simulink model "vector2"  (R2020a)
settings: Solver=FixedStepDiscrete  StartTime=0.0  StopTime=10.0  FixedStep=1  RelTol=1e-3
libraries: simulink x5, hdlsllib x3
settings Model: Creator=cyarp  LastModifiedBy=cyarp

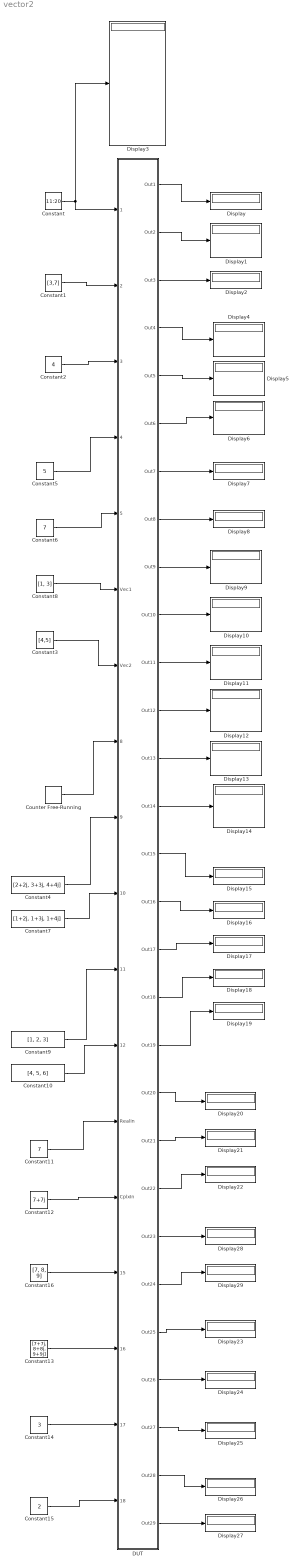
== system vector2 ==
  Constant : Constant  Value=11:20
  Constant1 : Constant  Value=[3,7]  OutDataTypeStr=int8
  Constant10 : Constant  Value=[4, 5, 6]
  Constant11 : Constant  Value=7
  Constant12 : Constant  Value=7+7j
  Constant13 : Constant  Value=[7+7j, 8+8j, 9+9j]
  Constant14 : Constant  Value=3  OutDataTypeStr=int8
  Constant15 : Constant  Value=2  OutDataTypeStr=int8
  Constant16 : Constant  Value=[7, 8, 9]
  Constant2 : Constant  Value=4  OutDataTypeStr=int8
  Constant3 : Constant  Value=[4,5]
  Constant4 : Constant  Value=[2+2j, 3+3j, 4+4j]
  Constant5 : Constant  Value=5
  Constant6 : Constant  Value=7
  Constant7 : Constant  Value=[1+2j, 1+3j, 1+4j]
  Constant8 : Constant  Value=[1, 3]
  Constant9 : Constant  Value=[1, 2, 3]
  Counter Free-Running : simulink/Sources/Counter Free-Running  NumBits=16  tsamp=-1
  DUT : Subsystem
  Display{,1..29} (30 alike) : Display
  wires:
  Constant/1 -> DUT/1(InVector), Display3/1
  Constant1/1 -> DUT/2(VecSelect)
  Constant2/1 -> DUT/3(ScalarSelect)
  Constant5/1 -> DUT/4(Scalar1)
  Constant6/1 -> DUT/5(Scalar2)
  Constant8/1 -> DUT/6(Vec1)
  Constant3/1 -> DUT/7(Vec2)
  Counter Free-Running/1 -> DUT/8(counter)
  Constant4/1 -> DUT/9(ComplVec1)
  Constant7/1 -> DUT/10(ComplVec2)
  Constant9/1 -> DUT/11(RealVec1)
  Constant10/1 -> DUT/12(RealVec2)
  Constant11/1 -> DUT/13(RealIn)
  Constant12/1 -> DUT/14(CplxIn)
  Constant13/1 -> DUT/16(ComplexCoef)
  Constant14/1 -> DUT/17(signed1)
  Constant15/1 -> DUT/18(signed2)
  DUT/1(Out1) -> Display/1
  DUT/2(Out2) -> Display1/1
  DUT/3(Out3) -> Display2/1
  DUT/4(Out4) -> Display4/1
  DUT/5(Out5) -> Display5/1
  DUT/6(Out6) -> Display6/1
  DUT/7(Out7) -> Display7/1
  DUT/8(Out8) -> Display8/1
  DUT/9(Out9) -> Display9/1
  DUT/10(Out10) -> Display10/1
  DUT/11(Out11) -> Display11/1
  DUT/12(Out12) -> Display12/1
  DUT/13(Out13) -> Display13/1
  DUT/14(Out14) -> Display14/1
  DUT/15(Out15) -> Display15/1
  DUT/16(Out16) -> Display16/1
  DUT/17(Out17) -> Display17/1
  DUT/18(Out18) -> Display18/1
  DUT/19(Out19) -> Display19/1
  DUT/20(Out20) -> Display20/1
  DUT/21(Out21) -> Display21/1
  DUT/22(Out22) -> Display22/1
  DUT/25(Out25) -> Display23/1
  DUT/26(Out26) -> Display24/1
  DUT/27(Out27) -> Display25/1
  DUT/28(Out28) -> Display26/1
  DUT/29(Out29) -> Display27/1
  DUT/23(Out23) -> Display28/1
  DUT/24(Out24) -> Display29/1
  Constant16/1 -> DUT/15(RealCoef)

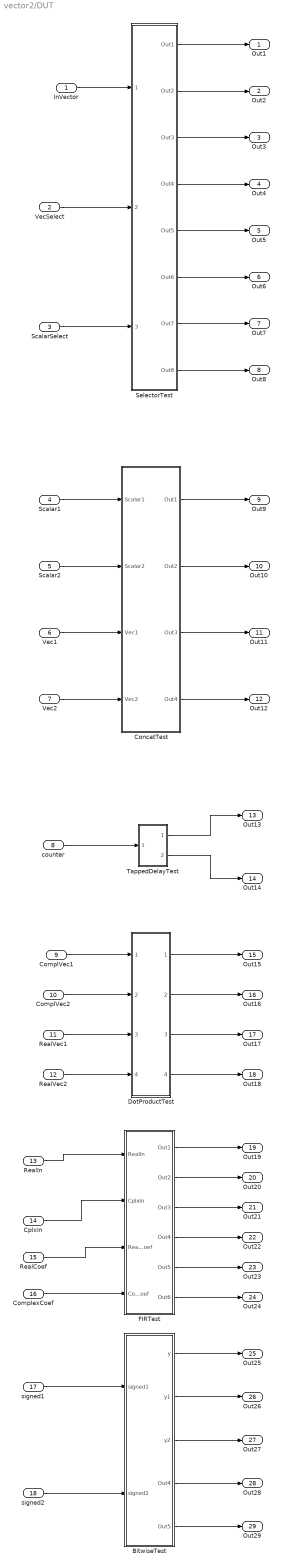
== system vector2/DUT ==
  InVector : Inport
  VecSelect : Inport  Port=2
  ScalarSelect : Inport  Port=3
  Scalar1 : Inport  Port=4
  Scalar2 : Inport  Port=5
  Vec1 : Inport  Port=6
  Vec2 : Inport  Port=7
  counter : Inport  Port=8
  ComplVec1 : Inport  Port=9
  ComplVec2 : Inport  Port=10
  RealVec1 : Inport  Port=11
  RealVec2 : Inport  Port=12
  RealIn : Inport  Port=13
  CplxIn : Inport  Port=14
  RealCoef : Inport  Port=15
  ComplexCoef : Inport  Port=16
  signed1 : Inport  Port=17
  signed2 : Inport  Port=18
  BitwiseTest : Subsystem
  ConcatTest : Subsystem
  DotProductTest : Subsystem
  FIRTest : Subsystem
  SelectorTest : Subsystem
  TappedDelayTest : Subsystem
  Out1 : Outport
  Out2 : Outport  Port=2
  Out3 : Outport  Port=3
  Out4 : Outport  Port=4
  Out5 : Outport  Port=5
  Out6 : Outport  Port=6
  Out7 : Outport  Port=7
  Out8 : Outport  Port=8
  Out9 : Outport  Port=9
  Out10 : Outport  Port=10
  Out11 : Outport  Port=11
  Out12 : Outport  Port=12
  Out13 : Outport  Port=13
  Out14 : Outport  Port=14
  Out15 : Outport  Port=15
  Out16 : Outport  Port=16
  Out17 : Outport  Port=17
  Out18 : Outport  Port=18
  Out19 : Outport  Port=19
  Out20 : Outport  Port=20
  Out21 : Outport  Port=21
  Out22 : Outport  Port=22
  Out23 : Outport  Port=23
  Out24 : Outport  Port=24
  Out25 : Outport  Port=25
  Out26 : Outport  Port=26
  Out27 : Outport  Port=27
  Out28 : Outport  Port=28
  Out29 : Outport  Port=29
  wires:
  RealIn/1 -> FIRTest/1(RealIn)
  FIRTest/1(Out1) -> Out19/1
  FIRTest/3(Out3) -> Out21/1
  SelectorTest/2(Out2) -> Out2/1
  FIRTest/4(Out4) -> Out22/1
  DotProductTest/2(Out2) -> Out16/1
  FIRTest/2(Out2) -> Out20/1
  DotProductTest/4(Out4) -> Out18/1
  ComplVec2/1 -> DotProductTest/2(ComplVec2)
  SelectorTest/1(Out1) -> Out1/1
  SelectorTest/3(Out3) -> Out3/1
  InVector/1 -> SelectorTest/1(InVector)
  ConcatTest/4(Out4) -> Out12/1
  SelectorTest/7(Out7) -> Out7/1
  counter/1 -> TappedDelayTest/1(In1)
  RealVec1/1 -> DotProductTest/3(RealVec1)
  ConcatTest/3(Out3) -> Out11/1
  VecSelect/1 -> SelectorTest/2(VecSelect)
  CplxIn/1 -> FIRTest/2(CplxIn)
  signed1/1 -> BitwiseTest/1(signed1)
  ScalarSelect/1 -> SelectorTest/3(ScalarSelect)
  SelectorTest/8(Out8) -> Out8/1
  BitwiseTest/1(y) -> Out25/1
  ComplexCoef/1 -> FIRTest/4(ComplexCoef)
  BitwiseTest/4(Out4) -> Out28/1
  SelectorTest/5(Out5) -> Out5/1
  ConcatTest/1(Out1) -> Out9/1
  Scalar2/1 -> ConcatTest/2(Scalar2)
  Vec1/1 -> ConcatTest/3(Vec1)
  SelectorTest/4(Out4) -> Out4/1
  DotProductTest/1(Out1) -> Out15/1
  signed2/1 -> BitwiseTest/2(signed2)
  ComplVec1/1 -> DotProductTest/1(ComplVec1)
  Vec2/1 -> ConcatTest/4(Vec2)
  DotProductTest/3(Out3) -> Out17/1
  BitwiseTest/5(Out5) -> Out29/1
  Scalar1/1 -> ConcatTest/1(Scalar1)
  BitwiseTest/2(y1) -> Out26/1
  ConcatTest/2(Out2) -> Out10/1
  RealVec2/1 -> DotProductTest/4(RealVec2)
  SelectorTest/6(Out6) -> Out6/1
  TappedDelayTest/2(Out2) -> Out14/1
  BitwiseTest/3(y2) -> Out27/1
  TappedDelayTest/1(Out1) -> Out13/1
  FIRTest/5(Out5) -> Out23/1
  FIRTest/6(Out6) -> Out24/1
  RealCoef/1 -> FIRTest/3(RealCoef)

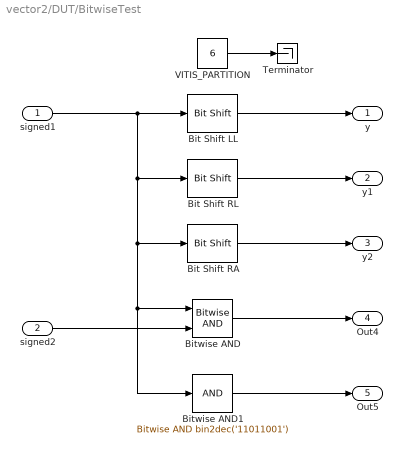
== system vector2/DUT/BitwiseTest ==
  signed1 : Inport
  signed2 : Inport  Port=2
  Bit Shift LL : hdlsllib/Logic and Bit Operations/Bit Shift  mode=Shift Left Logical  N=1
  Bit Shift RA : hdlsllib/Logic and Bit Operations/Bit Shift  mode=Shift Right Arithmetic  N=1
  Bit Shift RL : hdlsllib/Logic and Bit Operations/Bit Shift  mode=Shift Right Logical  N=1
  Bitwise AND : simulink/Logic and Bit Operations/Bitwise Operator  logicop=AND  UseBitMask=off  NumInputPorts=2  BitMask=bin2dec('11011001')  BitMaskRealWorld=Stored Integer
  Bitwise AND1 : simulink/Logic and Bit Operations/Bitwise Operator  logicop=AND  UseBitMask=on  BitMask=bin2dec('11011001')  BitMaskRealWorld=Stored Integer
  Terminator : Terminator
  VITIS_PARTITION : Constant  Value=6
  y : Outport
  y1 : Outport  Port=2
  y2 : Outport  Port=3
  Out4 : Outport  Port=4
  Out5 : Outport  Port=5
  wires:
  Bitwise AND1/1 -> Out5/1
  signed2/1 -> Bitwise AND/2
  Bitwise AND/1 -> Out4/1
  Bit Shift LL/1 -> y/1
  Bit Shift RA/1 -> y2/1
  Bit Shift RL/1 -> y1/1
  signed1/1 -> Bitwise AND1/1, Bitwise AND/1, Bit Shift RA/1, Bit Shift RL/1, Bit Shift LL/1
  VITIS_PARTITION/1 -> Terminator/1

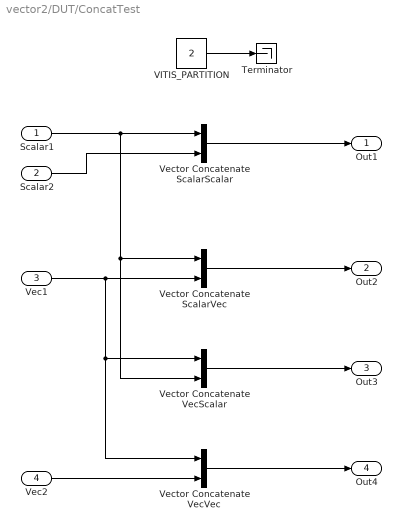
== system vector2/DUT/ConcatTest ==
  Scalar1 : Inport
  Scalar2 : Inport  Port=2
  Vec1 : Inport  Port=3
  Vec2 : Inport  Port=4
  Terminator : Terminator
  VITIS_PARTITION : Constant  Value=2
  Vector Concatenate ScalarScalar : Concatenate
  Vector Concatenate ScalarVec : Concatenate
  Vector Concatenate VecScalar : Concatenate
  Vector Concatenate VecVec : Concatenate
  Out1 : Outport
  Out2 : Outport  Port=2
  Out3 : Outport  Port=3
  Out4 : Outport  Port=4
  wires:
  Scalar2/1 -> Vector Concatenate ScalarScalar/2
  Vector Concatenate VecVec/1 -> Out4/1
  Vec2/1 -> Vector Concatenate VecVec/2
  Vector Concatenate ScalarScalar/1 -> Out1/1
  Scalar1/1 -> Vector Concatenate VecScalar/2, Vector Concatenate ScalarVec/1, Vector Concatenate ScalarScalar/1
  Vector Concatenate ScalarVec/1 -> Out2/1
  Vec1/1 -> Vector Concatenate VecVec/1, Vector Concatenate VecScalar/1, Vector Concatenate ScalarVec/2
  Vector Concatenate VecScalar/1 -> Out3/1
  VITIS_PARTITION/1 -> Terminator/1

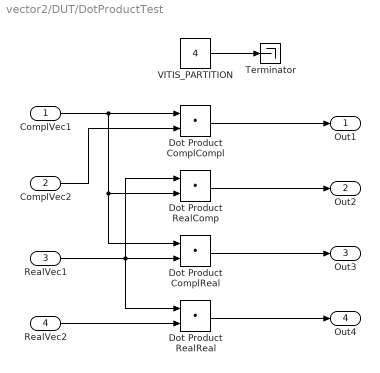
== system vector2/DUT/DotProductTest ==
  ComplVec1 : Inport
  ComplVec2 : Inport  Port=2
  RealVec1 : Inport  Port=3
  RealVec2 : Inport  Port=4
  Dot Product ComplCompl : DotProduct  InputSameDT=on  OutDataTypeStr=Inherit: Inherit via internal rule
  Dot Product ComplReal : DotProduct  InputSameDT=on  OutDataTypeStr=Inherit: Inherit via internal rule
  Dot Product RealComp : DotProduct  InputSameDT=on  OutDataTypeStr=Inherit: Inherit via internal rule
  Dot Product RealReal : DotProduct  InputSameDT=on  OutDataTypeStr=Inherit: Inherit via internal rule
  Terminator : Terminator
  VITIS_PARTITION : Constant  Value=4
  Out1 : Outport
  Out2 : Outport  Port=2
  Out3 : Outport  Port=3
  Out4 : Outport  Port=4
  wires:
  Dot Product ComplCompl/1 -> Out1/1
  Dot Product RealComp/1 -> Out2/1
  ComplVec2/1 -> Dot Product ComplCompl/2
  ComplVec1/1 -> Dot Product ComplReal/1, Dot Product RealComp/2, Dot Product ComplCompl/1
  RealVec2/1 -> Dot Product RealReal/2
  Dot Product ComplReal/1 -> Out3/1
  Dot Product RealReal/1 -> Out4/1
  RealVec1/1 -> Dot Product RealComp/1, Dot Product RealReal/1, Dot Product ComplReal/2
  VITIS_PARTITION/1 -> Terminator/1

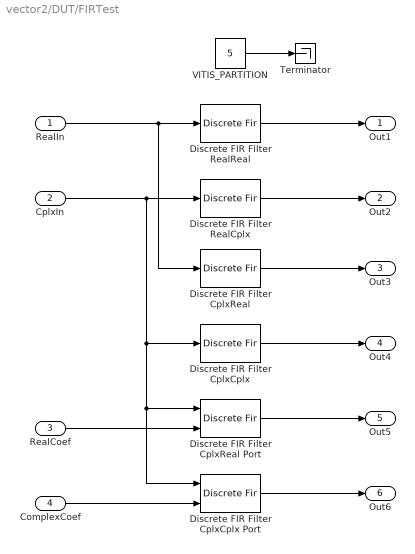
== system vector2/DUT/FIRTest ==
  RealIn : Inport
  CplxIn : Inport  Port=2
  RealCoef : Inport  Port=3
  ComplexCoef : Inport  Port=4
  Discrete FIR Filter CplxCplx : DiscreteFir  Coefficients=[0.5 0.5+0.5j 0.2]
  Discrete FIR Filter CplxCplx Port : DiscreteFir  CoefSource=Input port  Coefficients=[0.5 0.5+0.5j 0.2]
      settings: InputPortMap=u0,u1
  Discrete FIR Filter CplxReal : DiscreteFir  Coefficients=[0.5 0.5+0.5j 0.2]
  Discrete FIR Filter CplxReal Port : DiscreteFir  CoefSource=Input port  Coefficients=[0.5 0.5+0.5j 0.2]
      settings: InputPortMap=u0,u1
  Discrete FIR Filter RealCplx : DiscreteFir  Coefficients=[0.5 0.5 0.2]
  Discrete FIR Filter RealReal : DiscreteFir  Coefficients=[0.5 0.5 0.2]
  Terminator : Terminator
  VITIS_PARTITION : Constant  Value=5
  Out1 : Outport
  Out2 : Outport  Port=2
  Out3 : Outport  Port=3
  Out4 : Outport  Port=4
  Out5 : Outport  Port=5
  Out6 : Outport  Port=6
  wires:
  CplxIn/1 -> Discrete FIR Filter CplxCplx Port/1, Discrete FIR Filter CplxReal Port/1, Discrete FIR Filter CplxCplx/1, Discrete FIR Filter RealCplx/1
  Discrete FIR Filter CplxReal/1 -> Out3/1
  Discrete FIR Filter RealCplx/1 -> Out2/1
  RealIn/1 -> Discrete FIR Filter CplxReal/1, Discrete FIR Filter RealReal/1
  Discrete FIR Filter RealReal/1 -> Out1/1
  Discrete FIR Filter CplxCplx/1 -> Out4/1
  ComplexCoef/1 -> Discrete FIR Filter CplxCplx Port/2
  VITIS_PARTITION/1 -> Terminator/1
  Discrete FIR Filter CplxReal Port/1 -> Out5/1
  Discrete FIR Filter CplxCplx Port/1 -> Out6/1
  RealCoef/1 -> Discrete FIR Filter CplxReal Port/2

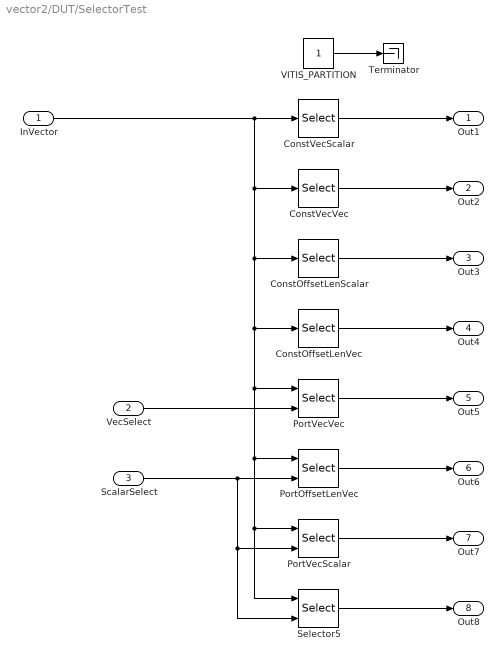
== system vector2/DUT/SelectorTest ==
  InVector : Inport
  VecSelect : Inport  Port=2
  ScalarSelect : Inport  Port=3
  ConstOffsetLenScalar : Selector  InputPortWidth=10  IndexOptions=Starting index (dialog)  Indices=3  OutputSizes=1
  ConstOffsetLenVec : Selector  InputPortWidth=10  IndexOptions=Starting index (dialog)  Indices=2  OutputSizes=3
  ConstVecScalar : Selector  InputPortWidth=10  IndexOptions=Index vector (dialog)  Indices=2  OutputSizes=3
  ConstVecVec : Selector  InputPortWidth=10  IndexOptions=Index vector (dialog)  Indices=[2,4]  OutputSizes=3
  PortOffsetLenVec : Selector  IndexMode=Zero-based  InputPortWidth=10  IndexOptions=Starting index (port)  Indices=2  OutputSizes=3
  PortVecScalar : Selector  IndexMode=Zero-based  InputPortWidth=10  IndexOptions=Index vector (port)  Indices=2  OutputSizes=3
  PortVecVec : Selector  IndexMode=Zero-based  InputPortWidth=10  IndexOptions=Index vector (port)  Indices=2  OutputSizes=3
  Selector5 : Selector  IndexMode=Zero-based  InputPortWidth=10  IndexOptions=Starting index (port)  Indices=2  OutputSizes=1
  Terminator : Terminator
  VITIS_PARTITION : Constant
  Out1 : Outport
  Out2 : Outport  Port=2
  Out3 : Outport  Port=3
  Out4 : Outport  Port=4
  Out5 : Outport  Port=5
  Out6 : Outport  Port=6
  Out7 : Outport  Port=7
  Out8 : Outport  Port=8
  wires:
  ConstOffsetLenVec/1 -> Out4/1
  PortVecScalar/1 -> Out7/1
  Selector5/1 -> Out8/1
  ConstVecScalar/1 -> Out1/1
  VecSelect/1 -> PortVecVec/2
  PortOffsetLenVec/1 -> Out6/1
  ConstOffsetLenScalar/1 -> Out3/1
  ConstVecVec/1 -> Out2/1
  PortVecVec/1 -> Out5/1
  ScalarSelect/1 -> Selector5/2, PortVecScalar/2, PortOffsetLenVec/2
  InVector/1 -> ConstVecVec/1, Selector5/1, PortVecScalar/1, PortOffsetLenVec/1, PortVecVec/1, ConstOffsetLenVec/1, ConstOffsetLenScalar/1, ConstVecScalar/1
  VITIS_PARTITION/1 -> Terminator/1

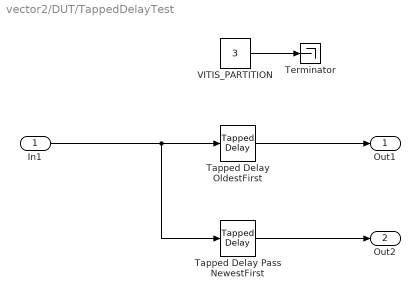
== system vector2/DUT/TappedDelayTest ==
  In1 : Inport
  Tapped Delay OldestFirst : simulink/Discrete/Tapped Delay  vinit=0.0  samptime=-1  NumDelays=3  DelayOrder=Oldest  includeCurrent=off
  Tapped Delay Pass NewestFirst : simulink/Discrete/Tapped Delay  vinit=0.0  samptime=-1  NumDelays=3  DelayOrder=Newest  includeCurrent=on
  Terminator : Terminator
  VITIS_PARTITION : Constant  Value=3
  Out1 : Outport
  Out2 : Outport  Port=2
  wires:
  Tapped Delay OldestFirst/1 -> Out1/1
  Tapped Delay Pass NewestFirst/1 -> Out2/1
  In1/1 -> Tapped Delay Pass NewestFirst/1, Tapped Delay OldestFirst/1
  VITIS_PARTITION/1 -> Terminator/1
